simulink model "Comunicacion_Arduino_2015"  (R2020a)
settings: Solver=VariableStepAuto  StartTime=0.0  StopTime=inf  RelTol=1e-3
undefined symbols (not defined in the file): LF, serial
libraries: instrumentlib x3
settings Model: Creator=Sergio  LastModifiedBy=HADOUNE
settings OptimizationCC: LifeSpan=inf
settings DebuggingCC: SFExecutionAtInitializationDiag=none  ArithmeticOperatorsInVariantConditions=warning
settings SFSimCC: CustomCodeUndefinedFunction=UseInterfaceOnly
settings CodeAppCC: StateflowObjectComments=on

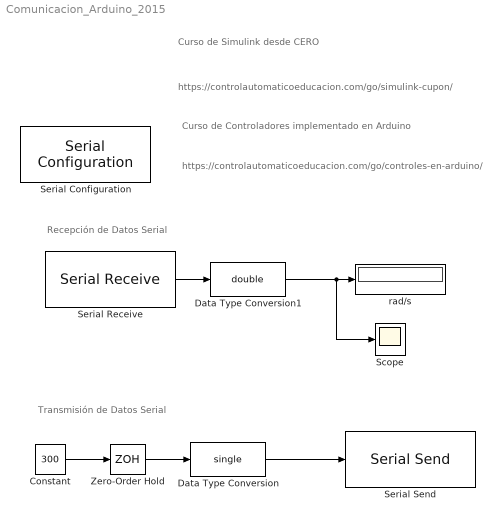
== system Comunicacion_Arduino_2015 ==
  note: Transmisión de Datos Serial
  note: Recepción de Datos Serial
  note: Curso de Simulink desde CERO
  note: https://controlautomaticoeducacion.com/go/simulink-cupon/
  note: https://controlautomaticoeducacion.com/go/controles-en-arduino/
  note: Curso de Controladores implementado en Arduino
  Constant : Constant  Value=300
  Data Type Conversion : DataTypeConversion  OutDataTypeStr=single
  Data Type Conversion1 : DataTypeConversion  OutDataTypeStr=double
  Scope : Scope
  Serial Configuration : instrumentlib/Serial Configuration  Priority=-200000  ComPortMenu=COM11  ComPort=COM11  ObjConstructor=serial('COM11');  BaudRate=9600  DataBits=8  Parity=none  StopBits=1  FlowControl=none  Timeout=10  ByteOrder=LittleEndian
  Serial Receive : instrumentlib/Serial Receive  Priority=1  ComPortMenu=COM11  ComPort=COM11  ObjConstructor=serial('COM11');  Header='V'  Terminator=LF ('\n')  DataSize=[1 1]  DataType=single  EnableBlockingMode=on  ActionDataUnavailable=Output last received value  CustomValue=0  SampleTime=0.04
  Serial Send : instrumentlib/Serial Send  Priority=1  ComPortMenu=COM11  ComPort=COM11  ObjConstructor=serial('COM11');  Terminator=<none>  EnableBlockingMode=on
  Zero-Order Hold : ZeroOrderHold  SampleTime=0.03
  rad/s : Display
  wires:
  Constant/1 -> Zero-Order Hold/1
  Zero-Order Hold/1 -> Data Type Conversion/1
  Data Type Conversion/1 -> Serial Send/1
  Serial Receive/1 -> Data Type Conversion1/1
  Data Type Conversion1/1 -> Scope/1, rad/s/1
